simulink model "storagesystemTFMvdefinitiva"  (R2016a)
settings: Solver=VariableStepAuto  StartTime=0.0  StopTime=10.0  MaxStep=1e-4  RelTol=1e-5
values from neighbouring files (symbols this model uses):
  Kp = 1.36    [Parameters_DC_Side_Voltage_Source.m]
  Ll = 0.0054    [Parameters_DC_Side_Voltage_Source.m]
  rl = 0.5    [Parameters_DC_Side_Voltage_Source.m]
  tau = 0.01    [Parameters_DC_Side_Voltage_Source.m]
  taupll = 0.0045    [Parameters_DC_Side_Voltage_Source.m]
libraries: powerlib x19, simulink x2, powerlib_meascontrol x1
settings Model: Creator=usuario  LastModifiedBy=usuario
settings DataIOCC: SaveFormat=StructureWithTime
settings DebuggingCC: AllowSymbolicDim=off
settings HardwareCC: ProdWordSize=32  ProdHWDeviceType=Specified

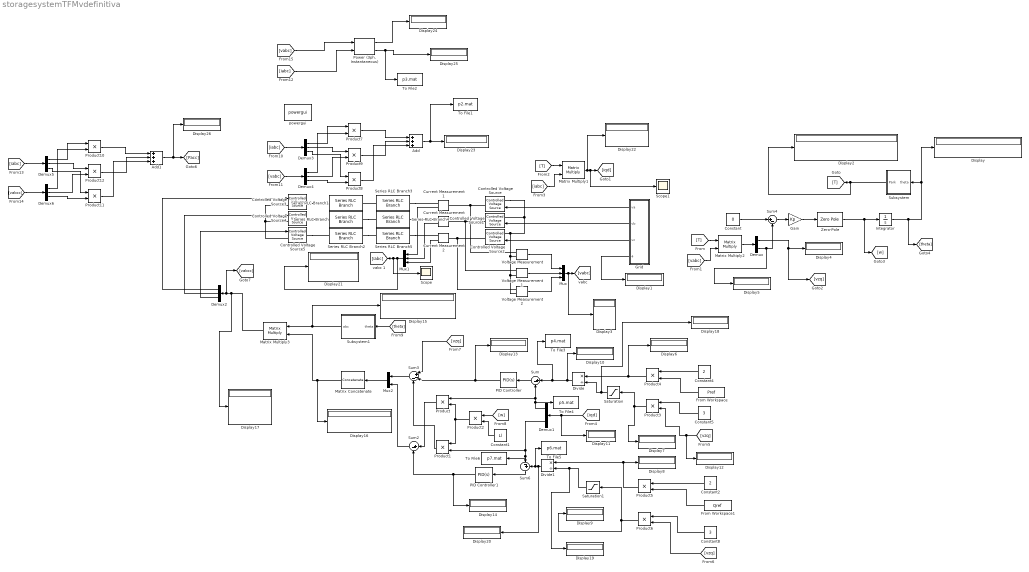
== system storagesystemTFMvdefinitiva ==
  Add : Sum  Inputs=+++
  Add1 : Sum  Inputs=+++
  Constant : Constant  Value=0
  Constant1 : Constant  Value=Ll
  Constant2 : Constant  Value=2
  Constant4 : Constant  Value=2
  Constant5 : Constant  Value=3
  Constant8 : Constant  Value=3
  Controlled Voltage Source{,1..5} (6 alike) : powerlib/Electrical Sources/Controlled Voltage Source  Initialize=on  Source_Type=AC  Amplitude=0  Phase=0  Frequency=0  Measurements=None
  Current Measurement : powerlib/Measurements/Current Measurement  PhasorSimulation=off  OutputType=Complex  PSBequivalent=0
  Current Measurement1 : powerlib/Measurements/Current Measurement  PhasorSimulation=off  OutputType=Complex  PSBequivalent=0
  Current Measurement2 : powerlib/Measurements/Current Measurement  PhasorSimulation=off  OutputType=Complex  PSBequivalent=0
  Demux : Demux  Outputs=2
  Demux1 : Demux  Outputs=2
  Demux{2..6} (5 alike) : Demux  Outputs=3
  Display{,1..26} (27 alike) : Display
  Divide : Product  Inputs=*/
  Divide1 : Product  Inputs=*/
  From Workspace : FromWorkspace  VariableName=Pref  SampleTime=0
  From Workspace1 : FromWorkspace  VariableName=Qref  SampleTime=0
  Gain : Gain  Gain=Kp
  "Grid " : Subsystem
  Integrator : Integrator
  Matrix Concatenate : Concatenate  NumInputs=1  Mode=Multidimensional array  ConcatenateDimension=2
  Matrix Multiply1 : Product  Multiplication=Matrix(*)
  Matrix Multiply2 : Product  Multiplication=Matrix(*)
  Matrix Multiply3 : Product  Multiplication=Matrix(*)
  Mux : Mux  Inputs=3
  Mux1 : Mux  Inputs=3
  Mux2 : Mux  Inputs=2
  PID Controller : simulink/Continuous/PID Controller  Controller=PID  TimeDomain=Continuous-time  SampleTime=-1  IntegratorMethod=Forward Euler  FilterMethod=Forward Euler  Form=Parallel  UseFilter=on  ControllerParametersSource=internal  P=Ll/tau  I=rl/tau  D=0  N=100  InitialConditionSource=internal  InitialConditionForIntegrator=0  InitialConditionForFilter=0  ExternalReset=none  LimitOutput=off  UpperSaturationLimit=inf  LowerSaturationLimit=-inf  LinearizeAsGain=on  AntiWindupMode=none  Kb=1  TrackingMode=off  Kt=1  PParamMin=[]  PParamMax=[]  IParamMin=[]  IParamMax=[]  DParamMin=[]  DParamMax=[]  NParamMin=[]  NParamMax=[]  KbParamMin=[]  KbParamMax=[]  KtParamMin=[]  KtParamMax=[]  POutMin=[]  POutMax=[]  IOutMin=[]  IOutMax=[]  DOutMin=[]  DOutMax=[]  NOutMin=[]  NOutMax=[]  KbOutMin=[]  KbOutMax=[]  KtOutMin=[]  KtOutMax=[]  IntegratorOutMin=[]  IntegratorOutMax=[]  FilterOutMin=[]  FilterOutMax=[]  SumOutMin=[]  SumOutMax=[]  SumI1OutMin=[]  SumI1OutMax=[]  SumI2OutMin=[]  SumI2OutMax=[]  SumI3OutMin=[]  SumI3OutMax=[]  SumDOutMin=[]  SumDOutMax=[]  SaturationOutMin=[]  SaturationOutMax=[]  IntegratorContinuousStateAttributes=''  IntegratorStateMustResolveToSignalObject=off  IntegratorRTWStateStorageClass=Auto  FilterContinuousStateAttributes=''  FilterStateMustResolveToSignalObject=off  FilterRTWStateStorageClass=Auto  DifferentiatorICPrevScaledInput=0  DifferentiatorOutMin=[]  DifferentiatorOutMax=[]
  PID Controller1 : simulink/Continuous/PID Controller  Controller=PID  TimeDomain=Continuous-time  SampleTime=-1  IntegratorMethod=Forward Euler  FilterMethod=Forward Euler  Form=Parallel  UseFilter=on  ControllerParametersSource=internal  P=Ll/tau  I=rl/tau  D=0  N=100  InitialConditionSource=internal  InitialConditionForIntegrator=0  InitialConditionForFilter=0  ExternalReset=none  LimitOutput=off  UpperSaturationLimit=inf  LowerSaturationLimit=-inf  LinearizeAsGain=on  AntiWindupMode=none  Kb=1  TrackingMode=off  Kt=1  PParamMin=[]  PParamMax=[]  IParamMin=[]  IParamMax=[]  DParamMin=[]  DParamMax=[]  NParamMin=[]  NParamMax=[]  KbParamMin=[]  KbParamMax=[]  KtParamMin=[]  KtParamMax=[]  POutMin=[]  POutMax=[]  IOutMin=[]  IOutMax=[]  DOutMin=[]  DOutMax=[]  NOutMin=[]  NOutMax=[]  KbOutMin=[]  KbOutMax=[]  KtOutMin=[]  KtOutMax=[]  IntegratorOutMin=[]  IntegratorOutMax=[]  FilterOutMin=[]  FilterOutMax=[]  SumOutMin=[]  SumOutMax=[]  SumI1OutMin=[]  SumI1OutMax=[]  SumI2OutMin=[]  SumI2OutMax=[]  SumI3OutMin=[]  SumI3OutMax=[]  SumDOutMin=[]  SumDOutMax=[]  SaturationOutMin=[]  SaturationOutMax=[]  IntegratorContinuousStateAttributes=''  IntegratorStateMustResolveToSignalObject=off  IntegratorRTWStateStorageClass=Auto  FilterContinuousStateAttributes=''  FilterStateMustResolveToSignalObject=off  FilterRTWStateStorageClass=Auto  DifferentiatorICPrevScaledInput=0  DifferentiatorOutMin=[]  DifferentiatorOutMax=[]
  "Power (3ph, Instantaneous)" : powerlib_meascontrol/Measurements/Power (3ph, Instantaneous)
  Product{,1..12} (13 alike) : Product
  Saturation : Saturate  UpperLimit=1000  LowerLimit=200
  Saturation1 : Saturate  UpperLimit=1000  LowerLimit=200
  Scope : Scope
  Scope1 : Scope
  Series RLC Branch : powerlib/Elements/Series RLC Branch  LConnTagsString=__new0  RConnTagsString=__new0  BranchType=R  Resistance=0.5  Inductance=1e-3  SetiL0=off  InitialCurrent=0  Capacitance=1e-6  Setx0=off  InitialVoltage=0  Measurements=None
  Series RLC Branch1 : powerlib/Elements/Series RLC Branch  LConnTagsString=__new0  RConnTagsString=__new0  BranchType=R  Resistance=0.5  Inductance=1e-3  SetiL0=off  InitialCurrent=0  Capacitance=1e-6  Setx0=off  InitialVoltage=0  Measurements=None
  Series RLC Branch2 : powerlib/Elements/Series RLC Branch  LConnTagsString=__new0  RConnTagsString=__new0  BranchType=R  Resistance=0.5  Inductance=1e-3  SetiL0=off  InitialCurrent=0  Capacitance=1e-6  Setx0=off  InitialVoltage=0  Measurements=None
  Series RLC Branch3 : powerlib/Elements/Series RLC Branch  LConnTagsString=__new0  RConnTagsString=__new0  BranchType=L  Resistance=1  Inductance=0.0054  SetiL0=off  InitialCurrent=0  Capacitance=1e-6  Setx0=off  InitialVoltage=0  Measurements=None
  Series RLC Branch4 : powerlib/Elements/Series RLC Branch  LConnTagsString=__new0  RConnTagsString=__new0  BranchType=L  Resistance=1  Inductance=0.0054  SetiL0=off  InitialCurrent=0  Capacitance=1e-6  Setx0=off  InitialVoltage=0  Measurements=None
  Series RLC Branch5 : powerlib/Elements/Series RLC Branch  LConnTagsString=__new0  RConnTagsString=__new0  BranchType=L  Resistance=1  Inductance=0.0054  SetiL0=off  InitialCurrent=0  Capacitance=1e-6  Setx0=off  InitialVoltage=0  Measurements=None
  Subsystem : Subsystem
  Subsystem1 : Subsystem
  Sum : Sum  Inputs=|+-
  Sum2 : Sum  Inputs=|+-
  Sum3 : Sum  Inputs=|+--
  Sum4 : Sum  Inputs=|+-
  Sum6 : Sum  Inputs=|-+
  To File1 : ToFile  Filename=p2.mat  MatrixName=Pz1
  To File2 : ToFile  Filename=p3.mat  MatrixName=Qz
  To File3 : ToFile  Filename=p4.mat  MatrixName=iqref
  To File4 : ToFile  Filename=p5.mat  MatrixName=iq
  To File5 : ToFile  Filename=p6.mat  MatrixName=idref
  To File6 : ToFile  Filename=p7.mat  MatrixName=id
  Voltage Measurement : powerlib/Measurements/Voltage Measurement  PhasorSimulation=off  OutputType=Complex  PSBequivalent=0
  Voltage Measurement1 : powerlib/Measurements/Voltage Measurement  PhasorSimulation=off  OutputType=Complex  PSBequivalent=0
  Voltage Measurement2 : powerlib/Measurements/Voltage Measurement  PhasorSimulation=off  OutputType=Complex  PSBequivalent=0
  Zero-Pole : ZeroPole  Zeros=[-1/taupll]  Poles=[0]
  powergui : powerlib/powergui  Priority=1  SimulationMode=Continuous  SolverType=Tustin/Backward Euler (TBE)  SampleTime=50e-6  frequency=60  SPID=off  DisableSnubberDevices=off  DisableRonSwitches=off  DisableVfSwitches=off  SwTol=0  DisplayEquations=off  Interpol=off  ExternalGateDelay=off  methode=off  Ts=10  FunctionMessages=off  echomessages=off  HookPort=off  EnableUseOfTLC=off  x0status=blocks  frequencyindice=0  Pbase=100e6  ErrMax=1e-4  Iterations=50  UnitsV=kV  UnitsW=MW  buscounter=0  RestoreLinks=warning  ResistiveCurrentMeasurement=off  Frange=[0:2:500]  Ylog=off  Xlog=on  ShowGrid=off  save=off  variable=ZData  structure=0  ZoomFFT=off  StartTime=0.0  cycles=1  DisplayStyle=1  fundamental=60  FreqAxis=off  MaxFrequency=1000  frequencyindicesteady=1  RmsSteady=1  display=off
  wires:
  Product/1 -> Sum2/1
  Constant/1 -> Sum4/1
  Subsystem/1(Park) -> Display2/1, [T]
  Sum4/1 -> Gain/1
  Gain/1 -> Zero-Pole/1
  Zero-Pole/1 -> [w], Integrator/1
  Integrator/1 -> [theta], Display/1, Subsystem/1(theta)
  Constant1/1 -> Product2/2
  Product2/1 -> Product1/1, Product/2
  Voltage Measurement1/1 -> Mux/2
  Voltage Measurement/1 -> Mux/1
  Voltage Measurement2/1 -> Mux/3
  Mux/1 -> Display3/1, [vabc]
  [T] -> Matrix Multiply2/1
  [vabc] -> Matrix Multiply2/2
  Matrix Multiply2/1 -> Demux/1
  Demux/2 -> Display5/1, Sum4/2
  Current Measurement2/1 -> Mux1/3
  Current Measurement/1 -> Mux1/2
  Current Measurement1/1 -> Mux1/1
  Mux1/1 -> Display21/1, Scope/1, [iabc]
  [T] -> Matrix Multiply1/1
  [iabc] -> Matrix Multiply1/2
  Matrix Multiply1/1 -> Scope1/1, [iqd], Display22/1
  "Grid "/1(va) -> Controlled Voltage Source/1
  "Grid "/2(vb) -> Controlled Voltage Source1/1
  "Grid "/3(vc) -> Controlled Voltage Source2/1
  Demux1/1 -> Sum/2, Product/1, To File4/1
  [iqd] -> Demux1/1, Display11/1
  Sum/1 -> PID Controller/1
  Demux1/2 -> To File6/1, Sum6/1, Product1/2
  Sum6/1 -> PID Controller1/1
  PID Controller1/1 -> Sum2/2, Display14/1
  Product1/1 -> Sum3/3
  PID Controller/1 -> Display13/1, Sum3/2
  Sum3/1 -> Mux2/1
  Sum2/1 -> Mux2/2
  Subsystem1/1(abc) -> Display15/1, Matrix Multiply3/1
  Matrix Multiply3/1 -> Display17/1, [vabcc], Demux2/1
  Demux2/1 -> Controlled Voltage Source3/1
  Demux2/2 -> Controlled Voltage Source4/1
  Demux2/3 -> Controlled Voltage Source5/1
  From Workspace/1 -> Product4/2
  Constant4/1 -> Product4/1
  Product4/1 -> Display6/1, Divide/1
  Constant5/1 -> Product3/1
  [vzq] -> Display12/1, Product3/2
  Divide/1 -> Display10/1, To File3/1, Sum/1
  Constant2/1 -> Product5/1
  From Workspace1/1 -> Product5/2
  Constant8/1 -> Product6/1
  [vzq] -> Product6/2
  Product5/1 -> Divide1/1, Display8/1
  Divide1/1 -> To File5/1, Sum6/2, Display20/1
  Mux2/1 -> Matrix Concatenate/1
  Matrix Concatenate/1 -> Display16/1, Matrix Multiply3/2
  "Grid "/4(grid angle) -> Display1/1
  Demux/1 -> [vzq], Display4/1
  Product3/1 -> Saturation/1, Display7/1
  Product6/1 -> Saturation1/1, Display9/1
  [vzq] -> Sum3/1
  [w] -> Product2/1
  [theta] -> Subsystem1/1(theta)
  Saturation1/1 -> Display19/1, Divide1/2
  Saturation/1 -> Display18/1, Divide/2
  [iabc] -> Demux3/1
  [vabc] -> Demux4/1
  Demux3/1 -> Product7/1
  Demux4/1 -> Product7/2
  Demux3/2 -> Product9/1
  Demux4/2 -> Product9/2
  Demux3/3 -> Product8/1
  Demux4/3 -> Product8/2
  Product7/1 -> Add/1
  Product9/1 -> Add/2
  Product8/1 -> Add/3
  Add/1 -> To File1/1, Display23/1
  [iabc] -> Demux5/1
  [vabcc] -> Demux6/1
  Demux5/1 -> Product10/1
  Demux6/1 -> Product10/2
  Demux5/2 -> Product12/1
  Demux6/2 -> Product12/2
  Demux5/3 -> Product11/1
  Demux6/3 -> Product11/2
  Product10/1 -> Add1/1
  Product12/1 -> Add1/2
  Product11/1 -> Add1/3
  Add1/1 -> Display26/1, [Pacc]
  [iabc] -> "Power (3ph, Instantaneous)"/2
  [vabc] -> "Power (3ph, Instantaneous)"/1
  "Power (3ph, Instantaneous)"/1 -> Display24/1
  "Power (3ph, Instantaneous)"/2 -> To File2/1, Display25/1
  connections:
  Controlled Voltage Source3/RConn1 -- Series RLC Branch1/LConn1
  Controlled Voltage Source4/RConn1 -- Series RLC Branch/LConn1
  Controlled Voltage Source5/RConn1 -- Series RLC Branch2/LConn1
  Series RLC Branch3/LConn1 -- Series RLC Branch1/RConn1
  Series RLC Branch/RConn1 -- Series RLC Branch4/LConn1
  Series RLC Branch2/RConn1 -- Series RLC Branch5/LConn1
  Controlled Voltage Source1/RConn1 -- Current Measurement/LConn1 -- Voltage Measurement1/LConn1
  Series RLC Branch3/RConn1 -- Current Measurement1/RConn1
  Controlled Voltage Source/RConn1 -- Voltage Measurement/LConn1 -- Current Measurement1/LConn1
  Series RLC Branch5/RConn1 -- Current Measurement2/RConn1
  Series RLC Branch4/RConn1 -- Current Measurement/RConn1
  Controlled Voltage Source2/RConn1 -- Current Measurement2/LConn1 -- Voltage Measurement2/LConn1
  Controlled Voltage Source/LConn1 -- Controlled Voltage Source2/LConn1 -- Voltage Measurement/LConn2 -- Voltage Measurement1/LConn2 -- Voltage Measurement2/LConn2 -- Controlled Voltage Source1/LConn1
  Controlled Voltage Source3/LConn1 -- Controlled Voltage Source4/LConn1 -- Controlled Voltage Source5/LConn1

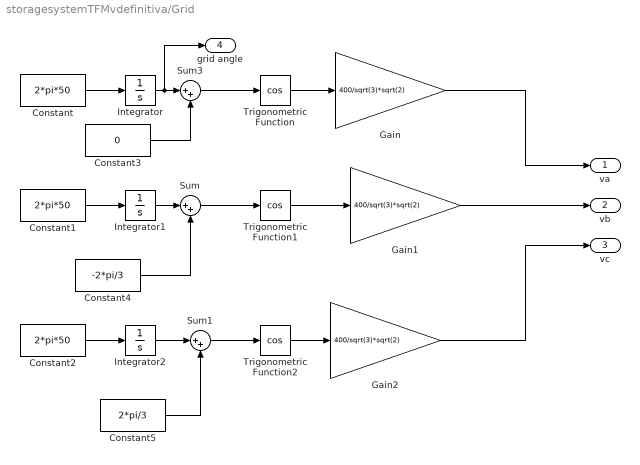
== system storagesystemTFMvdefinitiva/Grid  ==
  Constant : Constant  Value=2*pi*50
  Constant1 : Constant  Value=2*pi*50
  Constant2 : Constant  Value=2*pi*50
  Constant3 : Constant  Value=0
  Constant4 : Constant  Value=-2*pi/3
  Constant5 : Constant  Value=2*pi/3
  Gain : Gain  Gain=400/sqrt(3)*sqrt(2)
  Gain1 : Gain  Gain=400/sqrt(3)*sqrt(2)
  Gain2 : Gain  Gain=400/sqrt(3)*sqrt(2)
  Integrator : Integrator
  Integrator1 : Integrator
  Integrator2 : Integrator
  Sum : Sum  Inputs=|++
  Sum1 : Sum  Inputs=|++
  Sum3 : Sum  Inputs=|++
  Trigonometric Function : Trigonometry  Operator=cos
  Trigonometric Function1 : Trigonometry  Operator=cos
  Trigonometric Function2 : Trigonometry  Operator=cos
  va : Outport
  vb : Outport  Port=2
  vc : Outport  Port=3
  grid angle : Outport  Port=4
  wires:
  Constant2/1 -> Integrator2/1
  Integrator2/1 -> Sum1/1
  Gain2/1 -> vc/1
  Sum1/1 -> Trigonometric Function2/1
  Sum3/1 -> Trigonometric Function/1
  Integrator/1 -> grid angle/1, Sum3/1
  Constant5/1 -> Sum1/2
  Constant4/1 -> Sum/2
  Integrator1/1 -> Sum/1
  Trigonometric Function/1 -> Gain/1
  Gain/1 -> va/1
  Constant1/1 -> Integrator1/1
  Trigonometric Function2/1 -> Gain2/1
  Constant/1 -> Integrator/1
  Constant3/1 -> Sum3/2
  Trigonometric Function1/1 -> Gain1/1
  Gain1/1 -> vb/1
  Sum/1 -> Trigonometric Function1/1

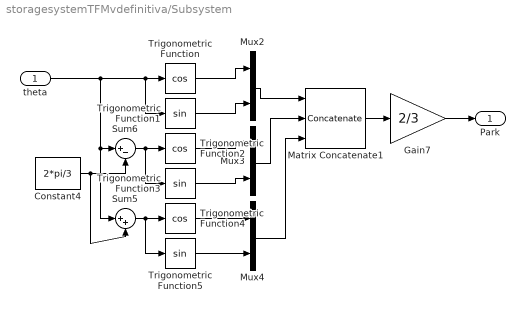
== system storagesystemTFMvdefinitiva/Subsystem ==
  theta : Inport  PortDimensions=1
  Constant4 : Constant  Value=2*pi/3  SampleTime=-1
  Gain7 : Gain  Gain=2/3
  Matrix Concatenate1 : Concatenate  NumInputs=3  Mode=Multidimensional array  ConcatenateDimension=2
  Mux2 : Mux  Inputs=2
  Mux3 : Mux  Inputs=2
  Mux4 : Mux  Inputs=2
  Sum5 : Sum  Inputs=|++
  Sum6 : Sum  Inputs=|+-
  Trigonometric Function : Trigonometry  Operator=cos
  Trigonometric Function1 : Trigonometry
  Trigonometric Function2 : Trigonometry  Operator=cos
  Trigonometric Function3 : Trigonometry
  Trigonometric Function4 : Trigonometry  Operator=cos
  Trigonometric Function5 : Trigonometry
  Park : Outport
  wires:
  Trigonometric Function/1 -> Mux2/1
  Sum5/1 -> Trigonometric Function4/1, Trigonometric Function5/1
  Trigonometric Function3/1 -> Mux3/2
  Trigonometric Function2/1 -> Mux3/1
  Sum6/1 -> Trigonometric Function2/1, Trigonometric Function3/1
  Trigonometric Function1/1 -> Mux2/2
  Gain7/1 -> Park/1
  Matrix Concatenate1/1 -> Gain7/1
  Mux4/1 -> Matrix Concatenate1/3
  Mux3/1 -> Matrix Concatenate1/2
  Mux2/1 -> Matrix Concatenate1/1
  Trigonometric Function5/1 -> Mux4/2
  Trigonometric Function4/1 -> Mux4/1
  Constant4/1 -> Sum6/2, Sum5/2
  theta/1 -> Sum5/1, Sum6/1, Trigonometric Function/1, Trigonometric Function1/1

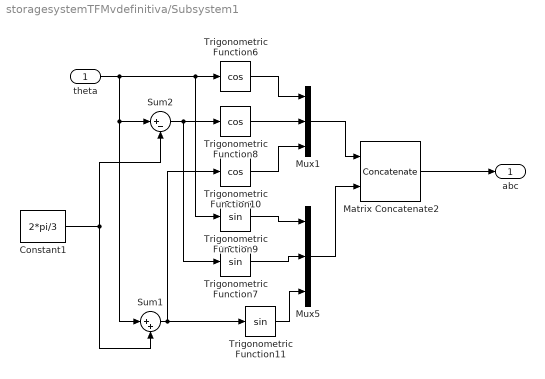
== system storagesystemTFMvdefinitiva/Subsystem1 ==
  theta : Inport  PortDimensions=1
  Constant1 : Constant  Value=2*pi/3  SampleTime=-1
  Matrix Concatenate2 : Concatenate  Mode=Multidimensional array  ConcatenateDimension=2
  Mux1 : Mux  Inputs=3
  Mux5 : Mux  Inputs=3
  Sum1 : Sum  Inputs=|++
  Sum2 : Sum  Inputs=|+-
  Trigonometric Function10 : Trigonometry  Operator=cos
  Trigonometric Function11 : Trigonometry
  Trigonometric Function6 : Trigonometry  Operator=cos
  Trigonometric Function7 : Trigonometry
  Trigonometric Function8 : Trigonometry  Operator=cos
  Trigonometric Function9 : Trigonometry
  abc : Outport
  wires:
  Trigonometric Function6/1 -> Mux1/1
  Sum1/1 -> Trigonometric Function10/1, Trigonometric Function11/1
  Sum2/1 -> Trigonometric Function7/1, Trigonometric Function8/1
  Mux1/1 -> Matrix Concatenate2/1
  Constant1/1 -> Sum2/2, Sum1/2
  theta/1 -> Trigonometric Function9/1, Trigonometric Function6/1, Sum2/1, Sum1/1
  Trigonometric Function11/1 -> Mux5/3
  Trigonometric Function9/1 -> Mux5/1
  Mux5/1 -> Matrix Concatenate2/2
  Trigonometric Function7/1 -> Mux5/2
  Matrix Concatenate2/1 -> abc/1
  Trigonometric Function8/1 -> Mux1/2
  Trigonometric Function10/1 -> Mux1/3
